simulink model "Car"  (R2021a)
settings: Solver=VariableStepAuto  StartTime=0.0  StopTime=10.0  RelTol=1e-3
libraries: sdl_lib x6, fl_lib x5, nesl_utility x3
settings Model: Creator=pdant  LastModifiedBy=pdant

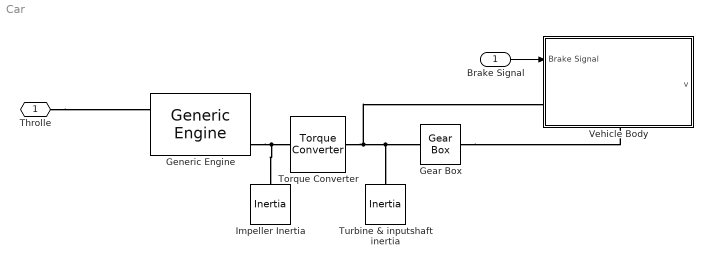
== system Car ==
  Brake Signal : Inport
  Gear Box : fl_lib/Mechanical/Mechanisms/Gear Box  ratio=5  t_in_specify=off  t_in_priority=None  t_in=0 N*m  t_in_nominal_specify=off  t_in_nominal_unit=N*m  t_in_nominal_value=1  t_out_specify=off  t_out_priority=None  t_out=0 N*m  t_out_nominal_specify=off  t_out_nominal_unit=N*m  t_out_nominal_value=1
  Generic Engine : sdl_lib/Engines & Motors/Generic Engine  model_parameterization=1  engine_type=1  P_max=150 kW  w_P_max=4500 rpm  w_max=8000 rpm  w_min=500 rpm  w_tab=[500, 1000, 2000, 3000, 4000, 5000, 6000, 7000] rpm  trq_tab=[380, 380, 380, 380, 350, 280, 200, 80] N*m  pwr_tab=[20, 40, 78, 120, 145, 148, 125, 60] kW  interp_method=simscape.enum.interpolation.linear  model_inertia=0  inertia=1 kg*m^2  initial_velocity=800 rpm  model_time_constant=0  time_constant=0.2 s  T0=0  w_thr=100 rpm  idle_speed=0  idle_speed_reference=1000 rpm  tau_controller=1 s  idle_w_thr=1 rpm  redline=0  redline_speed=5000 rpm  tau_redline=1 s  redline_w_thr=1 rpm  fc_model=0  fc_per_rev=25 mg/rev  displaced_volume=400 cm^3  rev_per_cycle=2  fc_w_tab=[1000, 2000, 3000, 4000, 5000, 6000] rpm  fc_trq_tab=[0, 80, 160, 200, 240, 320, 360, 400] N*m  fc_tab=[.5, .9, 1.4, 1.6, 1.9, 2.7, 3.4, 4.4; 1, 1.7, 2.7, 3.1, 3.6, 5, 6, 7.4; 1.4, 2.7, 4, 4.8, 5.6, 7.5, 8.5, 10.5; 2, 3.6, 5.8, 6.7, 8, 10.4, 11.7, 13.3; 2.5, 4.8, 7.9, 9.4, 10.8, 14, 16.2, 18.6; 3.1, 6, 10.3, 11.9, 13.8, 18.4, 22, 26.5] g/s  bmep_tab=[0, 250, 500, 625, 750, 1000, 1150, 1250] kPa  bsfc_tab=[410, 380, 300, 280, 270, 290, 320, 380; 410, 370, 290, 270, 260, 270, 285, 320; 415, 380, 290, 275, 265, 270, 270, 300; 420, 390, 310, 290, 285, 280, 280, 285; 430, 410, 340, 320, 310, 300, 310, 320; 450, 430, 370, 340, 330, 330, 350, 380] g/hr/kW  fc_interp_method=simscape.enum.interpolation.linear
      settings: SourceProductBaseCode=LD  InternalSimscapePortConfiguration="{\"Bottom\":[],\"Left\":[{\"id\":\"T\",\"label\":\"T\",\"type\":\"input\"},{\"id\":\"B\",\"label\":\"B\",\"type\":\"foundation.mechanical.rotational.rotational\"}],\"Right\":[{\"id\":\"P\",\"label\":\"P\",\"type\":\"output\"},{\"id\":\"FC\",\"label\":\"FC\",\"type\":\"output\"},{\"id\":\"F\",\"label\":\"F\",\"type\":\"foundation.mechanical.rotational.rotational\"}],\"Top\":[]}"
  Impeller Inertia : fl_lib/Mechanical/Rotational Elements/Inertia  inertia=0.01 kg*m^2  num_ports=foundation.enum.numPorts2.one  w_specify=off  w_priority=High  w=0 rad/s  w_nominal_specify=off  w_nominal_unit=rad/s  w_nominal_value=1  t_specify=off  t_priority=None  t=0 N*m  t_nominal_specify=off  t_nominal_unit=N*m  t_nominal_value=1
  Torque Converter : sdl_lib/Couplings & Drives/Torque Converter  coast_mode_modeling=sdl.enum.torqueConverterContinuousTwomode.twomode  SR_drive_tlu=[0, .5, .6, .7, .8, .87, .92, .94, .96, .97, 1]  TR_drive_tlu=[2.232, 1.5462, 1.4058, 1.2746, 1.1528, 1.0732, 1.0192, 1, 1, 1, 1]  CF_drive_tlu=1e-4 * [.72558, .66322, .63463, .59042, .51331, .4144, .29287, .22444, .12186, .04386, 0] m*N/rpm^2  SR_coast_tlu=[0, .5, .6, .7, .8, .87, .92, .94, .96, .97, 1]  CF_coast_tlu=1e-4 * [.5079, .4643, .4442, .4133, .3593, .2901, .205, .1571, .0853, .0307, 0] m*N/rpm^2  interp_method_twomode=simscape.enum.interpolation.linear  extrap_method_twomode=simscape.enum.extrapolation.linear  iniMode=sdl.enum.torqueConverterInitialMode.drive  delta_w=1 rpm  n_vector=[0, .5, .6, .7, .8, .87, .92, .94, .96, .97]  trq_vector=[2.232, 1.5462, 1.4058, 1.2746, 1.1528, 1.0732, 1.0192, .9983, .9983, .9983]  cf_vector_parameterization=sdl.enum.torqueConverterCFParameterization.SpeedToSqrtTorque  cf_vector_reference_speed=sdl.enum.torqueConverterCFReferenceSpeed.ImpellerSpeedAlways  cf_vector=[12.2938, 12.8588, 13.1452, 13.6285, 14.6163, 16.2675, 19.3503, 22.1046, 29.9986, 50] (rad/s)/(N*m)^0.5  cf_vector_sq=1e-3 * [6.616, 6.048, 5.787, 5.384, 4.681, 3.779, 2.671, 2.047, 1.111, .4] N*m/(rad/s)^2  interp_method_continuous=simscape.enum.interpolation.linear  extrap_method_continuous=simscape.enum.extrapolation.linear  model_lag=sdl.enum.torqueConverterLagOnOff.LagOff  tau=.02 s  initial_trq_ratio=0
      settings: SourceProductBaseCode=LD  InternalSimscapePortConfiguration="{\"Bottom\":[],\"Left\":[{\"id\":\"I\",\"label\":\"I\",\"type\":\"foundation.mechanical.rotational.rotational\"}],\"Right\":[{\"id\":\"T\",\"label\":\"T\",\"type\":\"foundation.mechanical.rotational.rotational\"}],\"Top\":[]}"
  Turbine & inputshaft inertia : fl_lib/Mechanical/Rotational Elements/Inertia  inertia=0.01 kg*m^2  num_ports=foundation.enum.numPorts2.one  w_specify=off  w_priority=High  w=0 rad/s  w_nominal_specify=off  w_nominal_unit=rad/s  w_nominal_value=1  t_specify=off  t_priority=None  t=0 N*m  t_nominal_specify=off  t_nominal_unit=N*m  t_nominal_value=1
  Vehicle Body : Subsystem
      settings: PortSchema="{\"entries\":[{\"content\":{\"sides\":[{\"content\":{\"connectorIds\":[\"In1\",\"LConn1\"]},\"type\":\"ConnectorPlacement.EquallySpacedRectSide\",\"uuid\":\"6403e31f-539e-4980-b9de-501066135396\"},{\"content\":{\"connectorIds\":[\"Out1\"],\"side\":\"RIGHT\"},\"type\":\"ConnectorPlacement.EquallySpacedRectSide\",\"uuid\":\"be935725-b53f-4529-96e3-3fd36410f394\"},{\"content\":{\"connectorIds\":[],\"side\":\"TOP\"},\"type\":\"ConnectorPlacement.EquallySpacedRectSide\",\"uuid\":\"39e0fc54-dd64-4cd9-96a2-10b656a79f52\"},{\"content\":{\"connectorIds\":[\"RConn1\"],\"side\":\"BOTTOM\"},\"type\":\"ConnectorPlacement.EquallySpacedRectSide\",\"uuid\":\"baa52323-f519-4b51-9bfa-229d4291b5ed\"}]},\"type\":\"ConnectorPlacement.EquallySpacedConnector\",\"uuid\":\"4dc9ab14-3c14-4c84-99b0-f606f907be91\"}],\"packageUris\":[\"http://schema.mathworks.com/mf0/Connector/R2020b\"],\"version\":\"1.0\"}"
  Throlle : PMIOPort  Side=Left
  wires:
  Brake Signal/1 -> Vehicle Body/1(Brake Signal)
  connections:
  Generic Engine/RConn3 -- Impeller Inertia/LConn1 -- Torque Converter/LConn1
  Torque Converter/RConn1 -- Vehicle Body/LConn1 -- Gear Box/LConn1 -- Turbine & inputshaft inertia/LConn1
  Throlle/RConn1 -- Generic Engine/LConn1
  Gear Box/RConn1 -- Vehicle Body/RConn1

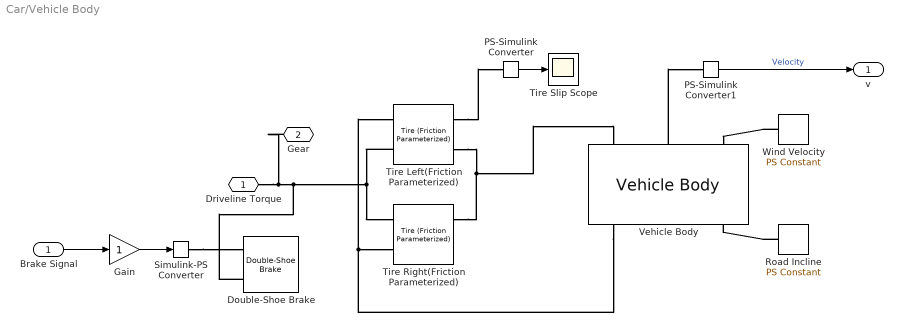
== system Car/Vehicle Body ==
  Brake Signal : Inport
  Double-Shoe Brake : sdl_lib/Brakes & Detents/Rotational/Double-Shoe Brake  r_drum=150 mm  r_act=100 mm  r_pin=125 mm  theta_pin=15 deg  theta_0=5 deg  theta_shoe=120 deg  mu_visc=.01 N*m/(rad/s)  thermal_port=simscape.enum.thermaleffects.omit  mu=0.3  temperature_TLU=[280, 300, 320] K  mu_TLU=[.1, .05, .03]  thermal_mass=50 kJ/K  w_thr=0.01 rad/s  enable_faults=simscape.enum.onoff.off  faulted_force=0 N  external_fault=simscape.enum.onoff.off  temporal_fault=simscape.enum.onoff.off  fault_time=5 s  report_fault=simscape.enum.assert.action.none  temperature_specify=off  temperature_priority=High  temperature=300 K  temperature_nominal_specify=off  temperature_nominal_unit=K  temperature_nominal_value=1
      settings: SourceProductBaseCode=LD  InternalSimscapePortConfiguration="{\"Bottom\":[],\"Left\":[{\"id\":\"F\",\"label\":\"F\",\"type\":\"input\"},{\"id\":\"S\",\"label\":\"S\",\"type\":\"foundation.mechanical.rotational.rotational\"}],\"Right\":[],\"Top\":[]}"
  Gain : Gain
  PS-Simulink Converter : nesl_utility/PS-Simulink Converter  PhysicalDomain=network_engine_domain  SubClassName=ps_output  LeftPortType=input  RightPortType=output  PseudoPeriodic=off  Frequencies=[]  Unit=inherit  AffineConversion=off
      settings: SourceProductBaseCode=PW,SS
  PS-Simulink Converter1 : nesl_utility/PS-Simulink Converter  PhysicalDomain=network_engine_domain  SubClassName=ps_output  LeftPortType=input  RightPortType=output  PseudoPeriodic=off  Frequencies=[]  Unit=inherit  AffineConversion=off
      settings: SourceProductBaseCode=PW,SS
  Road Incline : fl_lib/Physical Signals/Sources/PS Constant  constant=1
  Simulink-PS Converter : nesl_utility/Simulink-PS Converter  PhysicalDomain=network_engine_domain  SubClassName=ps_input  LeftPortType=input  RightPortType=output  PseudoPeriodic=off  Frequencies=[]  NoiseDistribution=none  NoiseParameters=[]  Unit=1  AffineConversion=off  FilteringAndDerivatives=provide  SimscapeFilterOrder=1  InputFilterTimeConstant=0.001  UdotUserProvided=0
      settings: SourceProductBaseCode=PW,SS
  Tire Left(Friction Parameterized) : sdl_lib/Tires & Vehicles/Tire (Friction Parameterized)  r_tire=0.3 m  friction_model=sdl.enum.friction_model_var.fixed  mu_static=0.90  mu_kinetic=0.70  slip_vector=[0, .02, .06, .15, .6, 1] rad/s  mu_kinetic_vector=[.89, .88, .8, .75, .7, .7]  interp_method=simscape.enum.interpolation.linear  extrap_method=simscape.enum.extrapolation.linear  model_compliance=0  stiffness=1e6 N/m  damping=1000 N/(m/s)  model_inertia=0  tire_inertia=1 kg*m^2  initial_velocity=0 rad/s  model_resistance=0  resistance_model=1  coeff=0.015  p_tire=250e3 Pa  alpha=-0.003  beta=0.97  coeff_a=84e-4  coeff_b=6.2e-4 s/m  coeff_c=1.6e-4 s^2/m^2  v_thr=0.001 m/s  v_tol=0.01 m/s  F_min=10 N  initial_traction_state=0
      settings: SourceProductBaseCode=LD  InternalSimscapePortConfiguration="{\"Bottom\":[],\"Left\":[{\"id\":\"N\",\"label\":\"N\",\"type\":\"input\"},{\"id\":\"A\",\"label\":\"A\",\"type\":\"foundation.mechanical.rotational.rotational\"}],\"Right\":[{\"id\":\"S\",\"label\":\"S\",\"type\":\"output\"},{\"id\":\"H\",\"label\":\"H\",\"type\":\"foundation.mechanical.translational.translational\"}],\"Top\":[]}"
  Tire Right(Friction Parameterized) : sdl_lib/Tires & Vehicles/Tire (Friction Parameterized)  r_tire=0.3 m  friction_model=sdl.enum.friction_model_var.fixed  mu_static=0.90  mu_kinetic=0.70  slip_vector=[0, .02, .06, .15, .6, 1] rad/s  mu_kinetic_vector=[.89, .88, .8, .75, .7, .7]  interp_method=simscape.enum.interpolation.linear  extrap_method=simscape.enum.extrapolation.linear  model_compliance=0  stiffness=1e6 N/m  damping=1000 N/(m/s)  model_inertia=0  tire_inertia=1 kg*m^2  initial_velocity=0 rad/s  model_resistance=0  resistance_model=1  coeff=0.015  p_tire=250e3 Pa  alpha=-0.003  beta=0.97  coeff_a=84e-4  coeff_b=6.2e-4 s/m  coeff_c=1.6e-4 s^2/m^2  v_thr=0.001 m/s  v_tol=0.01 m/s  F_min=10 N  initial_traction_state=0
      settings: SourceProductBaseCode=LD  InternalSimscapePortConfiguration="{\"Bottom\":[],\"Left\":[{\"id\":\"N\",\"label\":\"N\",\"type\":\"input\"},{\"id\":\"A\",\"label\":\"A\",\"type\":\"foundation.mechanical.rotational.rotational\"}],\"Right\":[{\"id\":\"S\",\"label\":\"S\",\"type\":\"output\"},{\"id\":\"H\",\"label\":\"H\",\"type\":\"foundation.mechanical.translational.translational\"}],\"Top\":[]}"
  Tire Slip Scope : Scope
  Vehicle Body : sdl_lib/Tires & Vehicles/Vehicle Body  mass=1200 kg  n_w=2  x_f=1.4 m  x_r=1.6 m  y_c=0.5 m  mass_var=simscape.enum.onoff.off  model_pitch=simscape.enum.onoff.off  inertia=4000 kg*m^2  suspension_model=sdl.enum.linearTLU.linear  k_f=1e4 N/m  b_f=1e4 N/(m/s)  k_r=1e4 N/m  b_r=1e4 N/(m/s)  k_f_TLU=[-2000, -1000, 0, 1000, 2000] N  x_f_TLU=[-.4, -.2, 0, .2, .4] m  b_f_TLU=[-200, -100, 0, 100, 200] N  v_f_TLU=[-4, -2, 0, 2, 4] m/s  k_r_TLU=[-2000, -1000, 0, 1000, 2000] N  x_r_TLU=[-.4, -.2, 0, .2, .4] m  b_r_TLU=[-200, -100, 0, 100, 200] N  v_r_TLU=[-4, -2, 0, 2, 4] m/s  interp_method=simscape.enum.interpolation.linear  extrap_method=simscape.enum.extrapolation.linear  model_hardstop=simscape.enum.onoff.off  upper_bound_f=.25 m  lower_bound_f=-.25 m  stop_k_f=1e6 N/m  stop_b_f=150 N/(m/s)  upper_bound_r=.25 m  lower_bound_r=-.25 m  stop_k_r=1e6 N/m  stop_b_r=150 N/(m/s)  initial_pitch=0 rad  initial_pitch_rate=0 rad/s  g=9.81 m/s^2  liftoff_warning=simscape.enum.onoff.off  area=3 m^2  Cd=0.4  rho=1.18 kg/m^3  v_specify=off  v_priority=High  v=0 m/s  v_nominal_specify=off  v_nominal_unit=m/s  v_nominal_value=1
  Wind Velocity : fl_lib/Physical Signals/Sources/PS Constant  constant=1
  Driveline Torque : PMIOPort  Side=Left
  Gear : PMIOPort  Port=2  Side=Right
  v : Outport
  wires:
  PS-Simulink Converter/1 -> Tire Slip Scope/1
  PS-Simulink Converter1/1 -> v/1  "Velocity"
  Gain/1 -> Simulink-PS Converter/1
  Brake Signal/1 -> Gain/1
  connections:
  Vehicle Body/RConn1 -- Tire Right(Friction Parameterized)/LConn1 -- Tire Left(Friction Parameterized)/LConn1
  Tire Left(Friction Parameterized)/RConn2 -- Tire Right(Friction Parameterized)/RConn2 -- Vehicle Body/LConn1
  Tire Left(Friction Parameterized)/LConn2 -- Gear/RConn1 -- Driveline Torque/RConn1 -- Double-Shoe Brake/LConn2 -- Tire Right(Friction Parameterized)/LConn2
  Tire Left(Friction Parameterized)/RConn1 -- PS-Simulink Converter/LConn1
  Vehicle Body/LConn2 -- PS-Simulink Converter1/LConn1
  Simulink-PS Converter/RConn1 -- Double-Shoe Brake/LConn1
  Road Incline/RConn1 -- Vehicle Body/RConn3
  Wind Velocity/RConn1 -- Vehicle Body/LConn3
